simulink model "MSFartoystyringRL"  (R2018b)
settings: Solver=ode23  StartTime=tstart  StopTime=tstop  RelTol=1e-3  EnableMultiTasking=on
values from neighbouring files (symbols this model uses):
  c = sqrt(cun*ur*n + cnn*n^2)    [msfartoystyring.m]    (also in pathfollowing.m = 1; run_task_2_6.m = 1)
  d1 = -0.0021    [init_controllers.m]
  d2 = 1.0377    [init_controllers.m]
  K = -0.0337    [init_controllers.m]
  Kd_heading = 3*lambda_heading    (= 0.3)    [init_controllers.m]
  Ki_heading = lambda_heading^3    (= 0.001)    [init_controllers.m]
  Ki_speed = lambda_speed^2    (= 0.09)    [init_controllers.m]
  Kp_heading = 3*lambda_heading^2    (= 0.03)    [init_controllers.m]
  Kp_speed = 2*lambda_speed    (= 0.6)    [init_controllers.m]
  m = 5550    [init_controllers.m]
  omega_n = 0.008    [init_controllers.m]
  omega_psi = 0.1    [init_controllers.m]
  p0 = [1500 500]    [pathfollowing.m]    (also in run_task_2_6.m)
  psi0 = 50*deg2rad    (= 0.872664625997)    [pathfollowing.m]    (also in run_task_2_6.m)
  Q = Q_out.data(:,:,:,end)    [ttk23assignment.m]
  r0 = 0    [pathfollowing.m]    (also in run_task_2_6.m)
  T = 62.6809    [init_controllers.m]
  tsamp = 10    [pathfollowing.m]    (also in run_task_2_6.m)
  u_r_0 = v0(1)    [pathfollowing.m]    (also in run_task_2_6.m)
  v0 = [6.63 0]'    [pathfollowing.m]    (also in run_task_2_6.m)
  zeta_c = 1    [init_controllers.m]
undefined symbols (not defined in the file or in its folder): i, msfartoystyring, WP
settings Model: ExtModeAutoUpdateStatusClock=off  Creator=christh  LastModifiedBy=Eier
settings SolverCC: ZeroCrossAlgorithm=Adaptive
settings DataIOCC: LimitDataPoints=on  SaveFormat=Array  SignalLoggingSaveFormat=ModelDataLogs
settings OptimizationCC: ExpressionDepthLimit=2147483647  InitFltsAndDblsToZero=on  LifeSpan=inf
settings DebuggingCC: UnderspecifiedInitializationDetection=Classic  MergeDetectMultiDrivingBlocksExec=none  IgnoredZcDiagnostic=none  SolverPrmCheckMsg=warning  FcnCallInpInsideContextMsg=warning  StateNameClashWarn=warning  SFUnexpectedBacktrackingDiag=warning  SFNoUnconditionalDefaultTransitionDiag=warning  SFExecutionAtInitializationDiag=none
settings HardwareCC: ProdBitPerPointer=32  ProdBitPerSizeT=32  ProdBitPerPtrDiffT=32  ProdLargestAtomicFloat=None  ProdIntDivRoundTo=Undefined  ProdEndianess=Unspecified  ProdWordSize=32  ProdHWDeviceType=32-bit Generic
settings ModelReferenceCC: PropagateSignalLabelsOutOfModel=off
settings SFSimCC: SimUseLocalCustomCode=off
settings RTWCC: RTWUseLocalCustomCode=off
settings CodeAppCC: StateflowObjectComments=on
settings GRTTargetCC: TargetLangStandard=C89/C90 (ANSI)  GeneratePreprocessorConditionals=Disable all  CombineOutputUpdateFcns=off  GRTInterface=on
settings ConfigComp: CovMetricSettings=dw  CovHtmlReporting=on  CovSaveCumulativeToWorkspaceVar=on  CovSaveSingleToWorkspaceVar=on  CovExternalEMLEnable=off

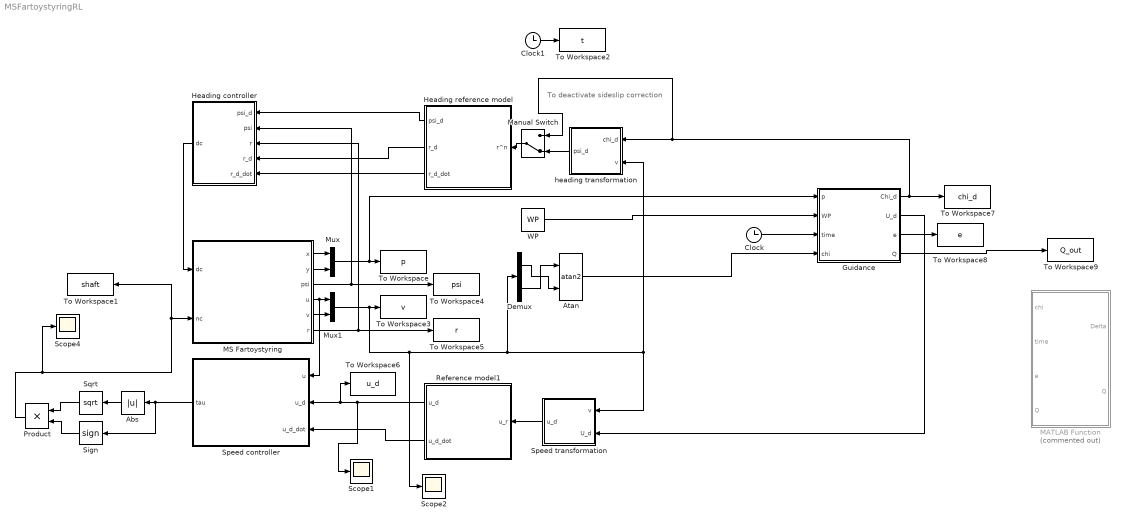
== system MSFartoystyringRL ==
  note: To deactivate sideslip correction
  Abs : Abs
  Atan : Trigonometry  Operator=atan2
  Clock : Clock
  Clock1 : Clock
  Demux : Demux  Outputs=2
  "Guidance " : Subsystem
  Heading controller : Subsystem
  Heading reference model : Subsystem
  MATLAB Function : MATLAB Function  Commented=on  TreatAsAtomicUnit=on
  MS Fartoystyring : Subsystem  mask(MS Fartoystyring for Assignment 3 G&C){x0=p0(1), y0=p0(2), u0=v0(1), v0=v0(2), psi0=psi0, r0=r0, c=c}
      mask prompts: x0 "x(t0) (m)"; y0 "y(t0) (m)"; u0 "u(t0) (m/s)"; v0 "v(t0) (m/s)"; psi0 "psi(t0) (rad)"; r0 "r(t0) (rad/s)"; c "current (0 or 1)"
      mask help:
      | Block corresponding to Figure 1 in the assignment text. Gives the response of the ship.
      |
      | The design speed of MS Fartoystyring is u=8.23 m/s.
      |
      | Input:
      | dc: commanded rudder (rad), dmax=25*pi/180
      | nc: commanded shaft speed (rad/s), nmax=85*2*pi/60
      |
      | Output:
      | x: north pos (m)
      | y: east pos (m)
      | u: surge (m/s)
      | v: sway (m/s)
      | psi: heading (rad)
      | r: yaw (rad/s)
      mask Help: Comments, bugs and help requests can be directed to the TA. Email on course website.
  Manual Switch : ManualSwitch  CurrentSetting=0
  Mux : Mux  Inputs=2
  Mux1 : Mux  Inputs=2
  Product : Product
  Reference model1 : Subsystem
  Scope1 : Scope
  Scope2 : Scope
  Scope4 : Scope
  Sign : Signum
  Speed controller : Subsystem
  Speed transformation : Subsystem
  Sqrt : Sqrt  SaturateOnIntegerOverflow=on
  To Workspace : ToWorkspace  VariableName=p  SampleTime=tsamp
  To Workspace1 : ToWorkspace  VariableName=shaft  SampleTime=tsamp
  To Workspace2 : ToWorkspace  VariableName=t  SampleTime=tsamp
  To Workspace3 : ToWorkspace  VariableName=v  SampleTime=tsamp
  To Workspace4 : ToWorkspace  VariableName=psi  SampleTime=tsamp
  To Workspace5 : ToWorkspace  VariableName=r  SampleTime=tsamp
  To Workspace6 : ToWorkspace  VariableName=u_d  SampleTime=tsamp
  To Workspace7 : ToWorkspace  VariableName=chi_d  SampleTime=tsamp
  To Workspace8 : ToWorkspace  VariableName=e  SampleTime=tsamp
  To Workspace9 : ToWorkspace  VariableName=Q_out  SaveFormat=Timeseries  SampleTime=-1
  WP : Constant  Value=WP
  heading transformation : Subsystem
  wires:
  MS Fartoystyring/1(x) -> Mux/1
  MS Fartoystyring/2(y) -> Mux/2
  MS Fartoystyring/4(u) -> Speed controller/1("u "), Mux1/1
  MS Fartoystyring/5(v) -> Mux1/2
  Mux/1 -> "Guidance "/1(p), To Workspace/1
  Clock1/1 -> To Workspace2/1
  Speed controller/1("tau ") -> Sign/1, Abs/1
  Abs/1 -> Sqrt/1
  Sign/1 -> Product/2
  Sqrt/1 -> Product/1
  Product/1 -> Scope4/1, To Workspace1/1, MS Fartoystyring/2(nc)
  Reference model1/1(u_d) -> Scope1/1, To Workspace6/1, Speed controller/2(u_d)
  Reference model1/2(u_d_dot) -> Speed controller/3(u_d_dot)
  WP/1 -> "Guidance "/2(WP)
  Heading reference model/2(r_d) -> Heading controller/4(r_d)
  MS Fartoystyring/6(r) -> Heading controller/3(r), To Workspace5/1
  MS Fartoystyring/3(psi) -> Heading controller/2(psi), To Workspace4/1
  Heading reference model/3("r_d_dot ") -> Heading controller/5("r_d_dot ")
  Mux1/1 -> Speed transformation/1("v "), heading transformation/2(v), Demux/1, Scope2/1, To Workspace3/1
  Heading controller/1(dc) -> MS Fartoystyring/1(dc)
  Heading reference model/1(psi_d) -> Heading controller/1(psi_d)
  "Guidance "/1("Chi_d ") -> To Workspace7/1, Manual Switch/1, heading transformation/1("chi_d ")
  "Guidance "/2(U_d) -> Speed transformation/2("U_d ")
  heading transformation/1("psi_d ") -> Manual Switch/2
  Speed transformation/1("u_d ") -> Reference model1/1(u_r)
  Manual Switch/1 -> Heading reference model/1(r^n)
  "Guidance "/3(e) -> To Workspace8/1
  Demux/2 -> Atan/1
  Demux/1 -> Atan/2
  Atan/1 -> "Guidance "/4(chi)
  Clock/1 -> "Guidance "/3("time ")
  "Guidance "/4(Q) -> To Workspace9/1

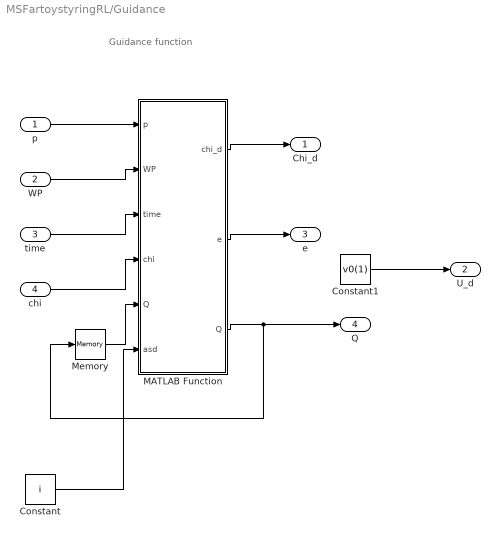
== system MSFartoystyringRL/Guidance  ==
  note: Guidance function
  p : Inport
  WP : Inport  Port=2
  "time " : Inport  Port=3
  chi : Inport  Port=4
  Constant : Constant  Value=i
  Constant1 : Constant  Value=v0(1)
  MATLAB Function : MATLAB Function  TreatAsAtomicUnit=on
  Memory : Memory  InitialCondition=Q
  "Chi_d " : Outport
  U_d : Outport  Port=2
  e : Outport  Port=3
  Q : Outport  Port=4
  wires:
  p/1 -> MATLAB Function/1(p)
  WP/1 -> MATLAB Function/2(WP)
  Constant1/1 -> U_d/1
  MATLAB Function/1(chi_d) -> "Chi_d "/1
  MATLAB Function/2(e) -> e/1
  "time "/1 -> MATLAB Function/3(time)
  MATLAB Function/3(Q) -> Memory/1, Q/1
  Memory/1 -> MATLAB Function/5("Q ")
  chi/1 -> MATLAB Function/4(chi)
  Constant/1 -> MATLAB Function/6(asd)

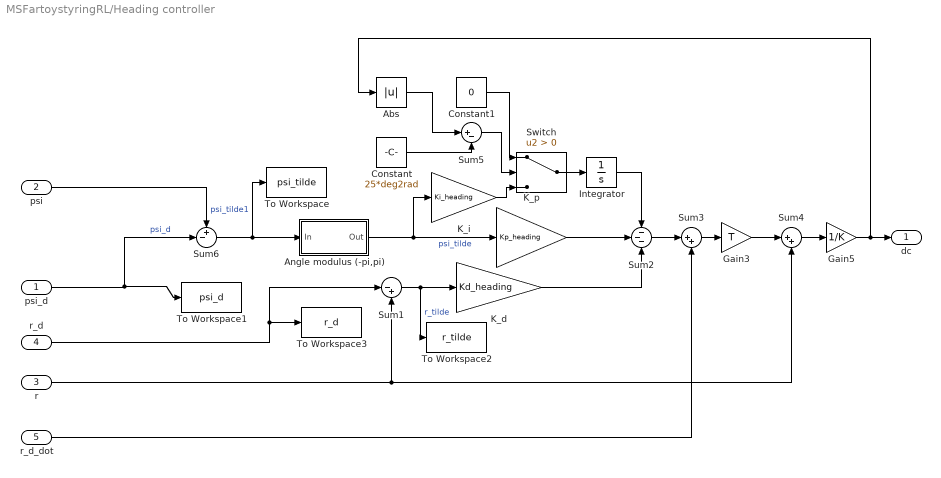
== system MSFartoystyringRL/Heading controller ==
  psi_d : Inport
  psi : Inport  Port=2
  r : Inport  Port=3
  r_d : Inport  Port=4
  "r_d_dot " : Inport  Port=5
  Abs : Abs
  Angle modulus (-pi,pi) : Subsystem
  Constant : Constant  Value=25*deg2rad
  Constant1 : Constant  Value=0
  Gain3 : Gain  Gain=T
  Gain5 : Gain  Gain=1/K
  Integrator : Integrator  LimitOutput=on  UpperSaturationLimit=deg2rad*25  LowerSaturationLimit=-deg2rad*25
  K_d : Gain  Gain=Kd_heading
  K_i : Gain  Gain=Ki_heading
  K_p : Gain  Gain=Kp_heading
  Sum1 : Sum  Inputs=|-+
  Sum2 : Sum  Inputs=---
  Sum3 : Sum  Inputs=|++
  Sum4 : Sum  Inputs=|++
  Sum5 : Sum  Inputs=|+-
  Sum6 : Sum  Inputs=+-|
  Switch : Switch  Criteria=u2 > Threshold
  To Workspace : ToWorkspace  VariableName=psi_tilde  SampleTime=tsamp
  To Workspace1 : ToWorkspace  VariableName=psi_d  SampleTime=tsamp
  To Workspace2 : ToWorkspace  VariableName=r_tilde  SampleTime=tsamp
  To Workspace3 : ToWorkspace  VariableName=r_d  SampleTime=tsamp
  dc : Outport
  wires:
  Sum1/1 -> To Workspace2/1, K_d/1  "r_tilde"
  Angle modulus (-pi,pi)/1(Out) -> K_p/1, K_i/1  "psi_tilde"
  K_p/1 -> Sum2/2
  Sum2/1 -> Sum3/1
  K_d/1 -> Sum2/3
  Sum3/1 -> Gain3/1
  Gain3/1 -> Sum4/1
  r/1 -> Sum4/2, Sum1/2
  Gain5/1 -> Abs/1, dc/1
  Sum4/1 -> Gain5/1
  Integrator/1 -> Sum2/1
  Abs/1 -> Sum5/1
  Sum5/1 -> Switch/2
  Constant/1 -> Sum5/2
  Constant1/1 -> Switch/1
  K_i/1 -> Switch/3
  Switch/1 -> Integrator/1
  psi_d/1 -> To Workspace1/1, Sum6/2  "psi_d"
  Sum6/1 -> To Workspace/1, Angle modulus (-pi,pi)/1(In)  "psi_tilde1"
  psi/1 -> Sum6/1
  "r_d_dot "/1 -> Sum3/2
  r_d/1 -> To Workspace3/1, Sum1/1

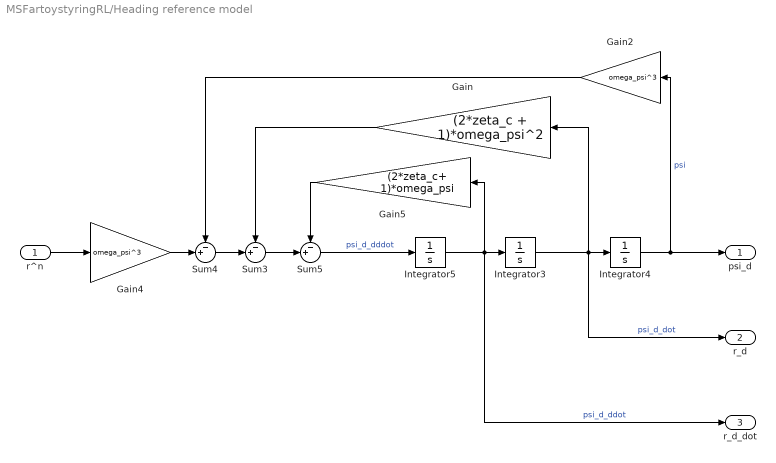
== system MSFartoystyringRL/Heading reference model ==
  r^n : Inport
  Gain : Gain  Gain=(2*zeta_c + 1)*omega_psi^2
  Gain2 : Gain  Gain=omega_psi^3
  Gain4 : Gain  Gain=omega_psi^3
  Gain5 : Gain  Gain=(2*zeta_c+ 1)*omega_psi
  Integrator3 : Integrator
  Integrator4 : Integrator  InitialCondition=psi0
  Integrator5 : Integrator
  Sum3 : Sum  Inputs=-+|
  Sum4 : Sum  Inputs=-+|
  Sum5 : Sum  Inputs=-+|
  psi_d : Outport
  r_d : Outport  Port=2
  "r_d_dot " : Outport  Port=3
  wires:
  Integrator3/1 -> r_d/1, Gain/1, Integrator4/1  "psi_d_dot"
  Gain/1 -> Sum3/1
  r^n/1 -> Gain4/1
  Integrator4/1 -> psi_d/1, Gain2/1  "psi"
  Sum4/1 -> Sum3/2
  Gain4/1 -> Sum4/2
  Sum3/1 -> Sum5/2
  Gain5/1 -> Sum5/1
  Sum5/1 -> Integrator5/1  "psi_d_dddot"
  Gain2/1 -> Sum4/1
  Integrator5/1 -> Gain5/1, "r_d_dot "/1, Integrator3/1  "psi_d_ddot"

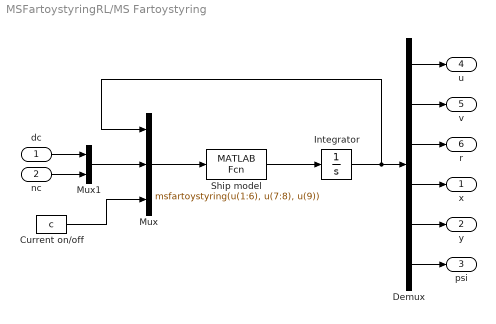
== system MSFartoystyringRL/MS Fartoystyring ==
  dc : Inport
  nc : Inport  Port=2
  Current on/off : Constant  Value=c
  Demux : Demux  Outputs=6
  Integrator : Integrator  InitialCondition=[u0 v0 r0 x0 y0 psi0]'
  Mux : Mux  Inputs=3
  Mux1 : Mux  Inputs=2
  Ship model : MATLABFcn  MATLABFcn=msfartoystyring(u(1:6), u(7:8), u(9))  OutputDimensions=6
  x : Outport
  y : Outport  Port=2
  psi : Outport  Port=3
  u : Outport  Port=4
  v : Outport  Port=5
  r : Outport  Port=6
  wires:
  Integrator/1 -> Mux/1, Demux/1
  Mux1/1 -> Mux/2
  dc/1 -> Mux1/1
  nc/1 -> Mux1/2
  Demux/1 -> u/1
  Demux/2 -> v/1
  Demux/3 -> r/1
  Demux/4 -> x/1
  Demux/5 -> y/1
  Demux/6 -> psi/1
  Ship model/1 -> Integrator/1
  Mux/1 -> Ship model/1
  Current on/off/1 -> Mux/3

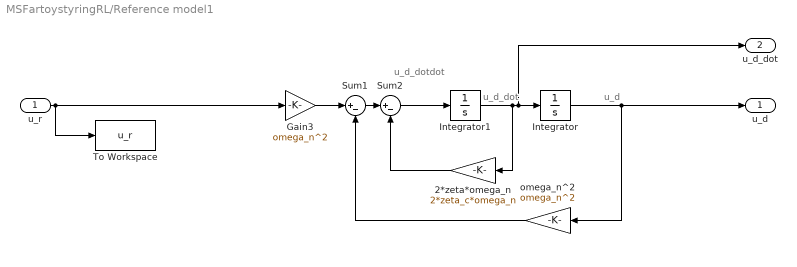
== system MSFartoystyringRL/Reference model1 ==
  note: u_d
  note: u_d_dot
  note: u_d_dotdot
  u_r : Inport
  2*zeta*omega_n : Gain  Gain=2*zeta_c*omega_n
  Gain3 : Gain  Gain=omega_n^2
  Integrator : Integrator  InitialCondition=u_r_0
  Integrator1 : Integrator
  Sum1 : Sum  Inputs=|+-
  Sum2 : Sum  Inputs=|+-
  To Workspace : ToWorkspace  VariableName=u_r  SampleTime=-1
  omega_n^2 : Gain  Gain=omega_n^2
  u_d : Outport
  u_d_dot : Outport  Port=2
  wires:
  Integrator1/1 -> 2*zeta*omega_n/1, Integrator/1, u_d_dot/1
  2*zeta*omega_n/1 -> Sum2/2
  Sum1/1 -> Sum2/1
  omega_n^2/1 -> Sum1/2
  Gain3/1 -> Sum1/1
  Sum2/1 -> Integrator1/1
  Integrator/1 -> omega_n^2/1, u_d/1
  u_r/1 -> To Workspace/1, Gain3/1

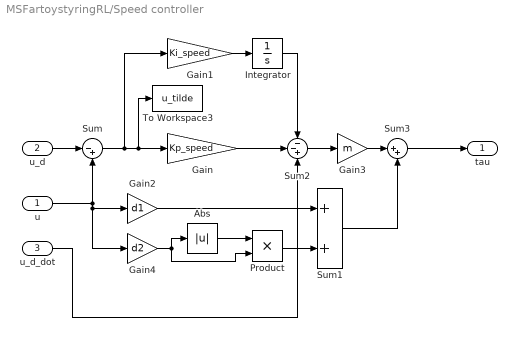
== system MSFartoystyringRL/Speed controller ==
  "u " : Inport
  u_d : Inport  Port=2
  u_d_dot : Inport  Port=3
  Abs : Abs
  Gain : Gain  Gain=Kp_speed
  Gain1 : Gain  Gain=Ki_speed
  Gain2 : Gain  Gain=d1
  Gain3 : Gain  Gain=m
  Gain4 : Gain  Gain=d2
  Integrator : Integrator
  Product : Product
  Sum : Sum  Inputs=|-+
  Sum1 : Sum
  Sum2 : Sum  Inputs=--+
  Sum3 : Sum  Inputs=|++
  To Workspace3 : ToWorkspace  VariableName=u_tilde  SampleTime=tsamp
  "tau " : Outport
  wires:
  Integrator/1 -> Sum2/1
  Gain/1 -> Sum2/2
  Sum2/1 -> Gain3/1
  Gain3/1 -> Sum3/1
  u_d_dot/1 -> Sum2/3
  Sum/1 -> To Workspace3/1, Gain/1, Gain1/1
  Gain1/1 -> Integrator/1
  u_d/1 -> Sum/1
  "u "/1 -> Gain4/1, Gain2/1, Sum/2
  Abs/1 -> Product/1
  Gain4/1 -> Abs/1, Product/2
  Gain2/1 -> Sum1/1
  Product/1 -> Sum1/2
  Sum1/1 -> Sum3/2
  Sum3/1 -> "tau "/1

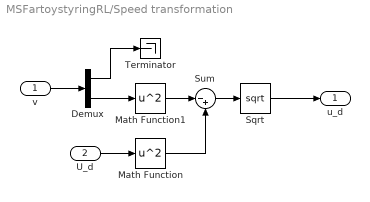
== system MSFartoystyringRL/Speed transformation ==
  "v " : Inport
  "U_d " : Inport  Port=2
  Demux : Demux  Outputs=2
  Math Function : Math  Operator=square  SaturateOnIntegerOverflow=on
  Math Function1 : Math  Operator=square  SaturateOnIntegerOverflow=on
  Sqrt : Sqrt  SaturateOnIntegerOverflow=on
  Sum : Sum  Inputs=|-+
  Terminator : Terminator
  "u_d " : Outport
  wires:
  "v "/1 -> Demux/1
  Sqrt/1 -> "u_d "/1
  "U_d "/1 -> Math Function/1
  Demux/1 -> Terminator/1
  Demux/2 -> Math Function1/1
  Math Function1/1 -> Sum/1
  Math Function/1 -> Sum/2
  Sum/1 -> Sqrt/1

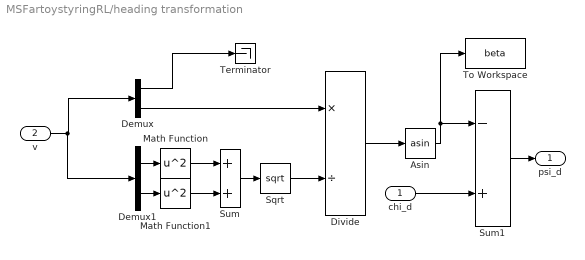
== system MSFartoystyringRL/heading transformation ==
  "chi_d " : Inport
  v : Inport  Port=2
  Asin : Trigonometry  Operator=asin
  Demux : Demux  Outputs=2
  Demux1 : Demux  Outputs=2
  Divide : Product  Inputs=*/
  Math Function : Math  Operator=square  SaturateOnIntegerOverflow=on
  Math Function1 : Math  Operator=square  SaturateOnIntegerOverflow=on
  Sqrt : Sqrt  SaturateOnIntegerOverflow=on
  Sum : Sum
  Sum1 : Sum  Inputs=-+
  Terminator : Terminator
  To Workspace : ToWorkspace  VariableName=beta  SampleTime=-1
  "psi_d " : Outport
  wires:
  v/1 -> Demux1/1, Demux/1
  Demux/1 -> Terminator/1
  Demux/2 -> Divide/1
  Demux1/1 -> Math Function/1
  Demux1/2 -> Math Function1/1
  Math Function/1 -> Sum/1
  Math Function1/1 -> Sum/2
  Sum/1 -> Sqrt/1
  Sqrt/1 -> Divide/2
  Divide/1 -> Asin/1
  Asin/1 -> To Workspace/1, Sum1/1
  "chi_d "/1 -> Sum1/2
  Sum1/1 -> "psi_d "/1

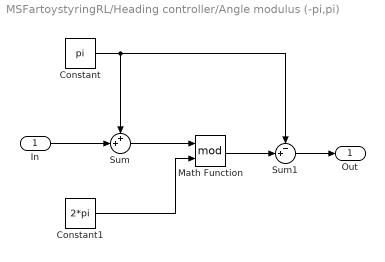
== system MSFartoystyringRL/Heading controller/Angle modulus (-pi,pi) ==
  In : Inport
  Constant : Constant  Value=pi
  Constant1 : Constant  Value=2*pi
  Math Function : Math  Operator=mod  SaturateOnIntegerOverflow=on
  Sum : Sum  Inputs=++|
  Sum1 : Sum  Inputs=-+|
  Out : Outport
  wires:
  Math Function/1 -> Sum1/2
  Sum/1 -> Math Function/1
  Constant/1 -> Sum1/1, Sum/1
  In/1 -> Sum/2
  Sum1/1 -> Out/1
  Constant1/1 -> Math Function/2

== matlab function MSFartoystyringRL/MATLAB Function ==
  data: chi input; time input; e input; Q input; Delta output; Q output
function [Delta, Q] = fcn(chi, time, e, Q)
R = @(x) x^2; %Simple reward function
%q-learning:
e_max = 1000; %Maximum cross-track error considered
de = 20; %Cross-track error threshold
dchi = deg2rad(10); %Course threshold
dt = 10; %Time step

epsilon = 0.3; %chance of picking random action
gamma = 0.9; %discount
alpha = 0.95; %learning rate

deltas = [100, 600, 1000]; %The three LOS-controller parameters this Q-learning algorithm will work with

persistent k;
if (isempty(k))
    k = 0;
end

chi = psi - alpha_k;

if floor(time/dt) >= k
    k = k + 1;
    %[e_tp, chi_tp] =sim(e_tp,chi_tp,a);
    %[e_tp, chi_tp] = run task 2_6 1 timestep with action a

    e_current = min(round(abs(e)/de), e_max)+1;
    chi_current = round(chi/dchi)+1;

    [value, a] = max(Q(e_current,chi_current,:));
    indices = find(Q(e_current,chi_current,:) == value);
    if (length(indices) > 1) || (rand() > epsilon)
        a = randi([1,3]);
    end

    Delta = deltas(a);
    
    Q(e_current, chi_current, a) = Q(e_current, chi_current, a)...
        + alpha*(R(e) + gamma*max(Q(e_next,chi_next,:)) - Q(e_current, chi_current, a));

end

== matlab function MSFartoystyringRL/Guidance /MATLAB Function ==
  settings: updateMethod=DISCRETE  sampleTime=tsamp
  data: p input; chi_d output; WP input; e output; time input; chi input; Q input; Q output; asd input
function [chi_d, e, Q] = fcn(p, WP, time, chi, Q, asd)
    
    %% FOR Q-LEARNING
    R = @(x) x^2; %Simple reward function, x will be the cross-track error going forward

    %Q-learning parameters:
    e_max = 1000; %Maximum cross-track error considered
    chi_max = 2*pi; %Maximum course value
    de = 20; %Cross-track error step-threshold
    dchi = deg2rad(10); %Course step-threshold
    dt = 10; %Time step
    
    e_greed = 0.3; %chance of picking random action instead of highest value
    gamma = 0.9; %discount
    alpha = 0.95; %learning rate

    deltas = [100, 600, 1000]; %The three LOS-vectors(the controller parameters) this Q-learning algorithm will switch between
                                %The goal is to find a switching behavior
                                %which performs better than a single,
                                %well-tuned controller.

    persistent j Delta e_prev chi_prev;  %Used to remember the LOS-vector(Delta), cross-track error
                                         % and course throughout the
                                         % simulink-loop
    if (isempty(j))
        j = 0;
    end
    if (isempty(Delta))
        Delta = 0;
    end
    if (isempty(e_prev))
        e_prev = 1;
    end
    if (isempty(chi_prev))
        chi_prev = 1;
    end

    %% GUIDANCE-block code from my old Guidance and Control-assignment
    %number of waypoints
    N = length(WP);

    % waypoint iteration
    persistent k;
    
    %waypoint iteration
    if (isempty(k))
        k = 1;
    end
    
    %reference waypoint
    xk_ref = WP(1, k);
    yk_ref = WP(2, k);
    
    %next waypoint
    xk_target = WP(1, k+1);
    yk_target = WP(2, k+1);
    
    
    if k ~= 6 && k ~= 1
        %calculating optimal turningradius
        lastWP = [WP(1,k-1); WP(2,k-1)];
        currentWP = [WP(1,k); WP(2,k)]; %way points
        nextWP = [WP(1,k+1); WP(2,k+1)];
        u = (lastWP - currentWP)/(norm(lastWP-currentWP));
        v = (nextWP - currentWP)/(norm(nextWP-currentWP)); %a,b,c
        w = (u + v)/(norm(u) + norm(v));
        a = acos((norm(v)^2 + norm(u+v)^2 - norm(u)^2)/(2*norm(v)*norm(u+v)));
        turningRadius = 900 / sin(a)*1.3;
    else
        turningRadius = 900*1.3;
    end
    
   
    alpha_k = atan2(yk_target-yk_ref, xk_target-xk_ref);
    
    Rp = [cos(alpha_k) -sin(alpha_k);
          sin(alpha_k) cos(alpha_k);];
      
    epsilon = Rp'*(p - [xk_ref yk_ref]');
    
    %R = sqrt(((xk_target-xk_ref)^2+(yk_target-yk_ref)^2))-epsilon(1,:); %Radius of acceptance
    chi_p = alpha_k;
    s = epsilon(1);
    e = epsilon(2);   %Cross-track error 

    %% Q LEARNING
    chi_pathrel = mod(chi + pi - alpha_k, 2*pi); %Course relative to the path between waypoints
    
    %Q-matrix update algorithm
    if floor(time/dt) >= j
        j = j + 1;
        %[e_tp, chi_tp] =sim(e_tp,chi_tp,a);
        %[e_tp, chi_tp] = run task 2_6 1 timestep with action a

        e_current = min(round(abs(e)/de), e_max/de)+1;  %The cross-track error's value will be =< e_max,
        chi_current = round((chi_pathrel)/dchi)+1;      % and both course and e are discretized to have each of their 
                                                        % step-values match the size of their respective Q-matrix indices

        [value, a] = max(Q(e_current,chi_current,:));   %Decides the best suited action(Delta) from Q,
        indices = find(Q(e_current,chi_current,:) == value);   % but will choose randomly if 2 or more
        if (length(indices) > 1) || (rand() < e_greed)         % actions are equal, or simply because
            a = randi([1,3]);                                  % the random exploration rolls high enough
        end

        Delta = deltas(a);       %Chooses the appropriate LOS-vector value depending on action a

        Q(e_prev, chi_prev, a) = Q(e_prev, chi_prev, a)...  %Updates Q's values for the next iteration
            + alpha*(R(e) + gamma*max(Q(e_current,chi_current,:)) - Q(e_prev, chi_prev, a));
        
        e_prev = e_current;
        chi_prev = chi_current;
    end
    %%
    chi_r = atan(-e/Delta);   %The controller using the various Delta-values
    chi_d = chi_p+chi_r;
    chi_d = mod(chi_d, 2*pi);
    
    
    if (norm(WP(:, k+1)-WP(:, k)) - s <= turningRadius) && (N-1 > k)
       k = k + 1;
    end
    
    
    
    
    
 
    [asd, time, e] %Debugging, shows which iteration, duration and current
    %cross-track error during training
end
